simulink model "RLE"  (Simulink 8.3)
settings: Solver=ode45  StartTime=0.0  StopTime=10.0  RelTol=1e-3
libraries: powerlib x13
settings Model: Creator=SUNIL YADAV  LastModifiedBy=SUNIL YADAV
settings DataIOCC: SignalLoggingSaveFormat=Dataset
settings DebuggingCC: UnderspecifiedInitializationDetection=Simplified  StateNameClashWarn=none
settings GRTTargetCC: CombineOutputUpdateFcns=on  GRTInterface=off

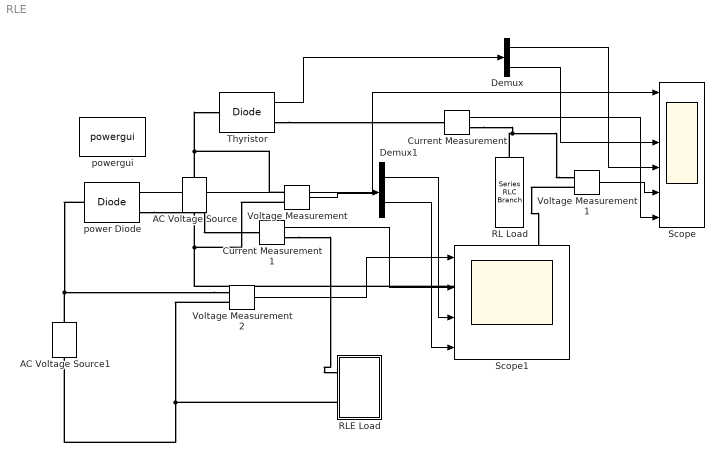
== system RLE ==
  AC Voltage Source : powerlib/Electrical Sources/AC Voltage Source  Amplitude=100  Phase=0  Frequency=60  SampleTime=0  Measurements=None
  AC Voltage Source1 : powerlib/Electrical Sources/AC Voltage Source  Amplitude=328  Phase=0  Frequency=50  SampleTime=0  Measurements=None
  Current Measurement : powerlib/Measurements/Current Measurement  PhasorSimulation=off  OutputType=Complex  PSBequivalent=0
  Current Measurement1 : powerlib/Measurements/Current Measurement  PhasorSimulation=off  OutputType=Complex  PSBequivalent=0
  Demux : Demux  Outputs=2
  Demux1 : Demux  Outputs=2
  RL Load : powerlib/Elements/Series RLC Branch  LConnTagsString=__new0  RConnTagsString=__new0  BranchType=RL  Resistance=1  Inductance=50e-3  SetiL0=off  InitialCurrent=0  Capacitance=1e-6  Setx0=off  InitialVoltage=0  Measurements=None
  RLE Load : Subsystem
  Scope : Scope  NumInputPorts=6
      settings: YMin=-100~-30~15~-5~-5~-5  YMax=100~100~28~5~5~5
  Scope1 : Scope  NumInputPorts=4
      settings: TimeRange=0.009770114942527997  YMin=-300~0~0~-275  YMax=350~13~12.5~25
  Thyristor : powerlib/Power Electronics/Diode  Ron=0.001  Lon=0  Vf=0.8  IC=0  UseSnubber=off  Rs=500  Cs=250e-9  Measurements=on
  Voltage Measurement : powerlib/Measurements/Voltage Measurement  PhasorSimulation=off  OutputType=Complex  PSBequivalent=0
  Voltage Measurement1 : powerlib/Measurements/Voltage Measurement  PhasorSimulation=off  OutputType=Complex  PSBequivalent=0
  Voltage Measurement2 : powerlib/Measurements/Voltage Measurement  PhasorSimulation=off  OutputType=Complex  PSBequivalent=0
  power Diode : powerlib/Power Electronics/Diode  Ron=0.001  Lon=0  Vf=0.8  IC=0  UseSnubber=off  Rs=500  Cs=250e-9  Measurements=on
  powergui : powerlib/powergui  Priority=1  SimulationMode=Discrete  SolverType=Tustin  SampleTime=50e-6  frequency=60  SPID=off  DisableSnubberDevices=off  DisableRonSwitches=off  DisableVfSwitches=off  SwTol=0  Interpol=off  DisplayEquations=off  Ts=0  methode=off  frequencyindice=50  Pbase=100e6  ErrMax=1e-4  Iterations=50  UnitsV=kV  UnitsW=MW  FunctionMessages=off  echomessages=off  HookPort=off  EnableUseOfTLC=off  x0status=blocks  RestoreLinks=warning  ResistiveCurrentMeasurement=off  Frange=[0:2:500]  Ylog=off  Xlog=on  ShowGrid=off  save=off  variable=ZData  structure=0  ZoomFFT=off  StartTime=0.0  cycles=1  DisplayStyle=1  fundamental=60  FreqAxis=off  MaxFrequency=1000  frequencyindicesteady=1  RmsSteady=1  display=off
  wires:
  Voltage Measurement/1 -> Scope/1
  Thyristor/1 -> Demux/1
  Demux/1 -> Scope/4
  Demux/2 -> Scope/3
  Voltage Measurement1/1 -> Scope/5
  Current Measurement/1 -> Scope/6
  Voltage Measurement2/1 -> Scope1/1
  Current Measurement1/1 -> Scope1/2
  Demux1/1 -> Scope1/3
  Demux1/2 -> Scope1/4
  power Diode/1 -> Demux1/1
  connections:
  Voltage Measurement/LConn1 -- AC Voltage Source/RConn1 -- Thyristor/LConn1
  Voltage Measurement1/LConn1 -- RL Load/LConn1 -- Current Measurement/RConn1
  Voltage Measurement1/LConn2 -- AC Voltage Source/LConn1 -- Voltage Measurement/LConn2
  Thyristor/RConn1 -- Current Measurement/LConn1
  Voltage Measurement2/LConn1 -- AC Voltage Source1/RConn1 -- power Diode/LConn1
  AC Voltage Source1/LConn1 -- Voltage Measurement2/LConn2 -- RLE Load/LConn2
  power Diode/RConn1 -- Current Measurement1/LConn1
  Current Measurement1/RConn1 -- RLE Load/LConn1

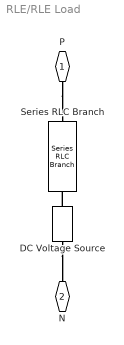
== system RLE/RLE Load ==
  DC Voltage Source : powerlib/Electrical Sources/DC Voltage Source  Amplitude=100  Measurements=None
  Series RLC Branch : powerlib/Elements/Series RLC Branch  LConnTagsString=__new0  RConnTagsString=__new0  BranchType=RL  Resistance=10  Inductance=100e-3  SetiL0=off  InitialCurrent=0  Capacitance=1e-6  Setx0=off  InitialVoltage=0  Measurements=None
  P : PMIOPort  Port=1  Side=Left
  " N" : PMIOPort  Port=2  Side=Left
  connections:
  DC Voltage Source/LConn1 -- " N"/RConn1
  P/RConn1 -- Series RLC Branch/LConn1
  DC Voltage Source/RConn1 -- Series RLC Branch/RConn1
